simulink model "final"  (R2020a)
settings: Solver=VariableStepAuto  StartTime=0.0  StopTime=5  RelTol=1e-3
undefined symbols (not defined in the file): fdesignblkfcn, gcbh
libraries: dspvision x6, dspfdesign x2, audiosources x1, dspsnks4 x1, dsparch4 x1, dspsrcs4 x1
settings Model: Creator=Karan  LastModifiedBy=Karan

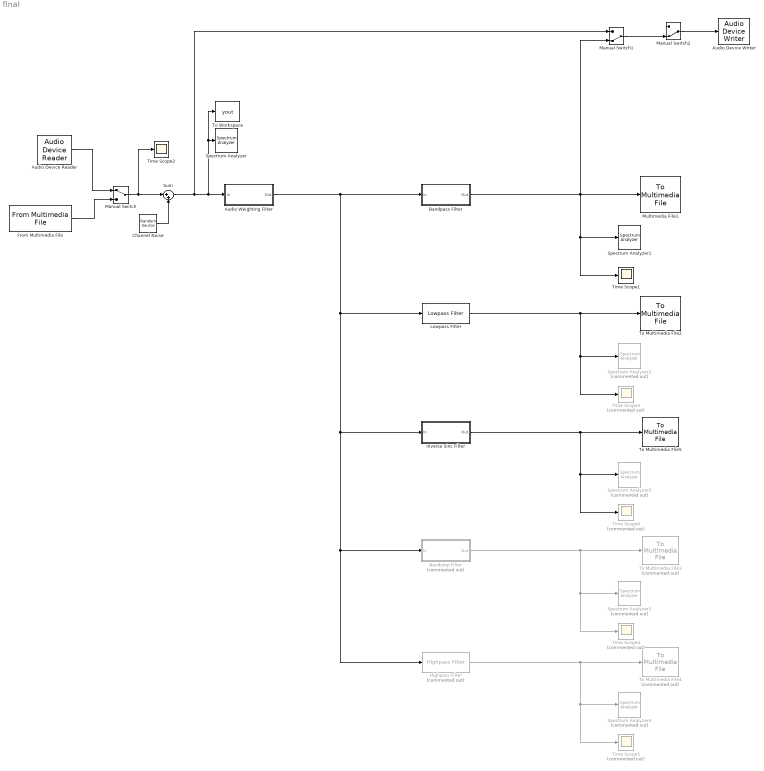
== system final ==
  Audio Device Reader : audiosources/Audio Device Reader  Driver=DirectSound  Device=Default  SampleRate=44100  NumChannels=1  SamplesPerFrame=1024  BitDepth=16-bit integer  NumBuffers=10  DefaultInputChannelMapping=on  InputChannelMapping=1:2  OutputNumOverrunSamples=off  OutputDataType=double  DriverIdx=1  DeviceWarnFlag=''
      settings: SourceProductBaseCode=AU
  Audio Device Writer : dspsnks4/Audio Device Writer  Driver=DirectSound  Device=Default  InheritSampleRate=on  SampleRate=44100  BitDepth=16-bit integer  BufferSize=4096  NumBuffers=10  DefaultOutputChannelMapping=on  OutputChannelMapping=1:2  OutputNumUnderrunSamples=off  DriverIdx=1  DeviceWarnFlag=''
  Audio Weighting Filter : Subsystem  DialogController=fdesignblkfcn  InitFcn=fdesignblkfcn(gcbh, {'InitFcn'});  mask(Audio Weighting Filter){}
      mask help: Design an audio weighting filter
      settings: CopyFcn=fdesignblkfcn(gcbh, {'CopyFcn'});
      mask Help: helpview(mapfilelocation('dsp'), 'dspaudioweightingfilter');
      mask Display: disp('Audio Weighting')
  Bandpass Filter : Subsystem  DialogController=fdesignblkfcn  InitFcn=fdesignblkfcn(gcbh, {'InitFcn'});  mask(Bandpass Filter){}
      mask help: Design a bandpass filter
      settings: CopyFcn=fdesignblkfcn(gcbh, {'CopyFcn'});
      mask Help: helpview(mapfilelocation('dsp'), 'dspbandpassfilter');
      mask Display: disp('Bandpass');
  Bandstop Filter : Subsystem  Commented=on  DialogController=fdesignblkfcn  InitFcn=fdesignblkfcn(gcbh, {'InitFcn'});  mask(Bandstop Filter){}
      mask help: Design a bandstop filter
      settings: CopyFcn=fdesignblkfcn(gcbh, {'CopyFcn'});
      mask Help: helpview(mapfilelocation('dsp'), 'dspbandstopfilter');
      mask Display: disp('Bandstop');
  Channel Noise : dspsrcs4/Random Source  SrcType=Gaussian  NormMethod=Ziggurat  CltLength=12  MinVal=0  MaxVal=1  MeanVal=0  VarVal=0.000005  RepMode=Not repeatable  rawSeed=1  IsInherit=off  SampMode=Discrete  SampTime=1/44100  SampFrame=1024  DataType=Double  OutComplex=Real  OutputFrames=off
  From Multimedia File : dspvision/From Multimedia File  inputFilename=D:\projects_on_github\tri-8_project\Matlab\dataset\noisy1.wav  readRange=[1 Inf]  loop=on  numPlays=inf  outputStreams=Audio only  videoDataType=single  audioDataType=double  inheritSampleTime=on  userDefinedSampleTime=1/30  noAudioOutput=off  isIntensityVideo=off  fourcc=RGB  colorVideoFormat=Separate color signals  outputEOF=off  dataOrg=Column-major  audioFrameSize=1024  computeAudioFrameSize=off  outSamplingMode=Sample based
  Highpass Filter : dspfdesign/Highpass Filter  Commented=on  FilterType=FIR  DesignForMinimumOrder=on  FilterOrder=50  StopbandFrequency=8e3  PassbandFrequency=12e3  StopbandAttenuation=80  PassbandRipple=0.1  InheritSampleRate=off  SampleRate=44100  SimulateUsing=Interpreted execution  roundingMode=Floor  coeffsDataTypeStr=fixdt(1,16)
  Inverse Sinc Filter : Subsystem  DialogController=fdesignblkfcn  InitFcn=fdesignblkfcn(gcbh, {'InitFcn'});  mask(Inverse Sinc Filter){}
      mask help: Design an inverse sinc filter
      settings: CopyFcn=fdesignblkfcn(gcbh, {'CopyFcn'});
      mask Help: helpview(mapfilelocation('dsp'), 'dspinversesincfilter');
      mask Display: disp('Inverse Sinc');
  Lowpass Filter : dspfdesign/Lowpass Filter  FilterType=FIR  DesignForMinimumOrder=on  FilterOrder=50  PassbandFrequency=3400  StopbandFrequency=6000  PassbandRipple=0.1  StopbandAttenuation=80  InheritSampleRate=off  SampleRate=44100  SimulateUsing=Interpreted execution  roundingMode=Floor  coeffsDataTypeStr=fixdt(1,16)
  Manual Switch : ManualSwitch
  Manual Switch1 : ManualSwitch  CurrentSetting=0
  Manual Switch2 : ManualSwitch  CurrentSetting=0
  Multimedia File1 : dspvision/To Multimedia File  outputFilename=D:\projects_on_github\tri-8_project\Matlab\BandPassOutput.wav  streamSelection=Audio only  videoCompressor=None (uncompressed)  audioCompressor=None (uncompressed)  imagePorts=Separate color signals  fileType=WAV  audioDatatype=16-bit integer  fourcc=RGB  videoQuality=75  mj2000CompFactor=10  mask(To Multimedia File){}
      mask Display: image('D:\projects_on_github\tri-8_project\icon.jfif'); % Use "Edit Image" on toolstrip to change.
  Spectrum Analyzer : SpectrumAnalyzer
  Spectrum Analyzer1 : SpectrumAnalyzer
  Spectrum Analyzer{2..5} (4 alike) : SpectrumAnalyzer  Commented=on
  Sum : Sum  Inputs=|++
  Time Scope1 : Scope
  Time Scope2 : Scope
  Time Scope{3..6} (4 alike) : Scope  Commented=on
  To Multimedia File2 : dspvision/To Multimedia File  outputFilename=D:\projects_on_github\tri-8_project\Matlab\LowPassOutput.wav  streamSelection=Audio only  videoCompressor=None (uncompressed)  audioCompressor=None (uncompressed)  imagePorts=Separate color signals  fileType=WAV  audioDatatype=16-bit integer  fourcc=RGB  videoQuality=75  mj2000CompFactor=10  mask(To Multimedia File){}
      mask Display: image('D:\projects_on_github\tri-8_project\icon.jfif'); % Use "Edit Image" on toolstrip to change.
  To Multimedia File3 : dspvision/To Multimedia File  Commented=on  outputFilename=D:\projects_on_github\tri-8_project\Matlab\BandStopOutput.wav  streamSelection=Audio only  videoCompressor=None (uncompressed)  audioCompressor=None (uncompressed)  imagePorts=Separate color signals  fileType=WAV  audioDatatype=16-bit integer  fourcc=RGB  videoQuality=75  mj2000CompFactor=10
  To Multimedia File4 : dspvision/To Multimedia File  Commented=on  outputFilename=D:\projects_on_github\tri-8_project\Matlab\HighPassOutput.wav  streamSelection=Audio only  videoCompressor=None (uncompressed)  audioCompressor=None (uncompressed)  imagePorts=Separate color signals  fileType=WAV  audioDatatype=16-bit integer  fourcc=RGB  videoQuality=75  mj2000CompFactor=10
  To Multimedia File5 : dspvision/To Multimedia File  outputFilename=D:\projects_on_github\tri-8_project\Matlab\InverseSincOutput.wav  streamSelection=Audio only  videoCompressor=None (uncompressed)  audioCompressor=None (uncompressed)  imagePorts=Separate color signals  fileType=WAV  audioDatatype=16-bit integer  fourcc=RGB  videoQuality=75  mj2000CompFactor=10  mask(To Multimedia File){}
      mask Display: image('D:\projects_on_github\tri-8_project\icon.jfif'); % Use "Edit Image" on toolstrip to change.
  To Workspace : ToWorkspace  VariableName=yout  SampleTime=-1
      settings: Save2DSignal=2-D array (concatenate along first dimension)
  wires:
  From Multimedia File/1 -> Manual Switch/2
  Audio Device Reader/1 -> Manual Switch/1
  Channel Noise/1 -> Sum/2
  Manual Switch/1 -> Time Scope2/1, Sum/1
  Lowpass Filter/1 -> Spectrum Analyzer2/1, Time Scope3/1, To Multimedia File2/1
  Bandstop Filter/1(Out) -> Spectrum Analyzer3/1, Time Scope4/1, To Multimedia File3/1
  Highpass Filter/1 -> Spectrum Analyzer4/1, Time Scope5/1, To Multimedia File4/1
  Sum/1 -> Manual Switch1/1, Audio Weighting Filter/1(In), To Workspace/1, Spectrum Analyzer/1
  Audio Weighting Filter/1(Out) -> Highpass Filter/1, Bandstop Filter/1(In), Inverse Sinc Filter/1(In), Lowpass Filter/1, Bandpass Filter/1(In)
  Bandpass Filter/1(Out) -> Manual Switch1/2, Multimedia File1/1, Spectrum Analyzer1/1, Time Scope1/1
  Inverse Sinc Filter/1(Out) -> Spectrum Analyzer5/1, Time Scope6/1, To Multimedia File5/1
  Manual Switch1/1 -> Manual Switch2/2
  Manual Switch2/1 -> Audio Device Writer/1

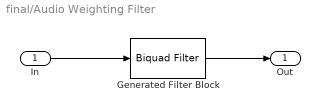
== system final/Audio Weighting Filter ==
  In : Inport
  Generated Filter Block : dsparch4/Biquad Filter  Tag=BlockMethodSubSystem  FilterSource=Dialog parameters  CoeffSource=Specify via dialog  FilterObject=BQF  IIRFiltStruct=Direct form II  BiQuadCoeffs=[0.000322318592897718971 0.000644637185795437942 0.000322318592897718971 1 -0.22455845805977917 0.0126066252715463997;1 -2 1 1 -1.89387049472307045 0.895159769094661439;1 -2 1 1 -1.99461445599302167 0.994621707014084477]  ScaleValues=[0.788048167211767292;1;1;922.43864463225691]  IC=0  ICnum=0  ICden=0  a0Flag=Warning  optimizeScaleValues=off  ScaleValueMode=Specify via input port (g)  InputProcessing=Columns as channels (frame based)  roundingMode=Floor  overflowMode=off  scaleValueFracLength=14  denProdOutputFracLength=30  denAccumFracLength=30  secondMemoryFracLength=15
  Out : Outport  VectorParamsAs1DForOutWhenUnconnected=off
  wires:
  In/1 -> Generated Filter Block/1
  Generated Filter Block/1 -> Out/1

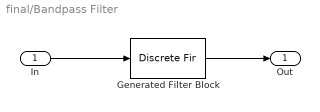
== system final/Bandpass Filter ==
  In : Inport
  Generated Filter Block : DiscreteFir  Tag=BlockMethodSubSystem  Coefficients=[-0.000844527152407708605 -0.000868562397225502948 -0.00116957293952449923 -0.00140352553207754964 -0.00150744965775681137 -0.00142845443379888918 -0.00113615100032245946 -0.000633399920489026349 3.8890998282847068e-05 0.000802430669925044394 0.00155053327984106849 0.00216334568785815553 0.00252906066623926869 0.00256430053522338887 0.0022313474523283929 0.00154779936195130279 0.000589010105671559014 -0.000522288015542289445 -0.00163619716288358297 -0.00260090540526047896 -0.00328662298843564573 -0.00361236887478878299 -0.00356005546849189926 -0.00317324951512466553 -0.00255473905797780603 -0.00183884524741045039 -0.00116989216351721611 -0.0006702717355624154 -0.000417805025534387635 -0.000430709163936836151 -0.000666023921114739566 -0.00103063604797135012 -0.00140285309979080227 -0.00166073040719528597 -0.00170975104047725937 -0.00150416142672811178 -0.00105705997801263459 -0.00043816865408110358 0.000242513896455011108 0.000859775723202255908 0.00130153535695951244 0.00149428225464512919 0.00142096258781483132 0.00112380329738751895 0.000695630323721911723 0.000258307321682619661 -6.65169364834449476e-05 -0.000184471009694367179 -5.22502422152739231e-05 0.000312808959320525664 0.000835725379946367281 0.00140171113245306581 0.00188290629102422571 0.0021687101586182209 0.00219279555742255905 0.00194960550536461309 0.0014967883978339602 0.000942467091606558711 0.000420688844749388829 5.9455733870843644e-05 -4.95874098292944614e-05 0.00012611843689524363 0.000551229383838804468 0.00112968550315262705 0.00172705058986454625 0.00220135626888997779 0.00243796013325304085 0.00237723221351059414 0.0020301515849451765 0.00147739859898147878 0.000851134737987892936 0.000304645405197287596 -2.45362664157255234e-05 -4.78931844306208036e-05 0.000251503798032808382 0.000813143385485723424 0.00151197185459038975 0.00218687423025305588 0.00267876041303893994 0.00286884600272527008 0.0027084843946502562 0.00223220324906475091 0.00155177460699580162 0.000830826586767605645 0.000246619686949600561 -5.25568822962958e-05 1.62854310485545643e-05 0.000448608883877401037 0.00115176008790661877 0.00196461380074925687 0.00269513061748809582 0.00316573559661484502 0.00325667292570079201 0.00293645872877977771 0.00227166552482126888 0.00141343803054731982 0.00056310351191782564 -7.53025250680251833e-05 -0.000344157009495414049 -0.000171780476247792164 0.000408022839556828969 0.0012612403531024061 0.00218361284411515595 0.00294781870362859685 0.00335822952789425208 0.00329883802248306891 0.00276364882401694805 0.00186096741407613042 0.000790494870982292133 -0.000202827515527535443 -0.000886470403153027551 -0.00109739540988425168 -0.000783030915458725958 -1.73930802721871426e-05 0.0010136082637835107 0.00205387967773256125 0.00283728196811974982 0.00315177869803649063 0.00289235940759398607 0.0020893396216802528 0.000905051665350609926 -0.000401866909465046639 -0.00153626562781204105 -0.00223704372134110553 -0.00234118477513825833 -0.00182637015731584949 -0.00082014067502192943 0.000426324760092775402 0.00159568661965235983 0.00237922054570370491 0.00255207910415520406 0.00203002271684176025 0.000894367368082263532 -0.000623077482255825644 -0.00219127628456664524 -0.00345756871074918851 -0.00413211362214908375 -0.00406036258673411754 -0.00326452265175293781 -0.0019437873571267225 -0.000431420107182345965 0.000881658006659412829 0.00164005892403595562 0.00161107111147124451 0.000745200775659432958 -0.000805996364953532034 -0.00271994083762002164 -0.00457588016984548755 -0.00595336149238870956 -0.00653452096578667051 -0.00618437479048854124 -0.00498998409671571816 -0.00324668708151827287 -0.00139387104974101109 8.68820925025471931e-05 0.000786909783874334824 0.000472575305548095486 -0.000852098204424628293 -0.00293738456659842391 -0.00533975824108989198 -0.00752207712372473473 -0.00898062826097165146 -0.00936845343587668078 -0.00858577816341373271 -0.00681354149649567205 -0.00448070355246299803 -0.00216977611076906406 -0.000481692636351701133 ...(+6520 chars)]  InputProcessing=Columns as channels (frame based)
  Out : Outport  VectorParamsAs1DForOutWhenUnconnected=off
  wires:
  In/1 -> Generated Filter Block/1
  Generated Filter Block/1 -> Out/1

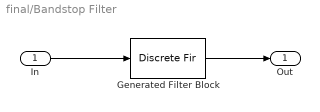
== system final/Bandstop Filter ==
  In : Inport
  Generated Filter Block : DiscreteFir  Tag=BlockMethodSubSystem  Coefficients=[-0.00049984690227566171 9.5100318056220678e-05 -0.018778888889125381 0.00020561736622238936 0.0019605411941885044 0.00023848464356614288 0.011427768692370117 0.00024928020776728103 -0.026344143468356181 0.00022323473160311075 0.033802321854574921 0.00024455404571586617 -0.019823660150560137 0.00024377045334422507 -0.019896328302992174 0.00022786848806407702 0.082714162332194516 0.00025656261277749384 -0.15101859373266049 0.00022072984516862497 0.20526035643478094 0.0002476136866061962 0.77489283142488197 0.0002476136866061962 0.20526035643478094 0.00022072984516862497 -0.15101859373266049 0.00025656261277749384 0.082714162332194516 0.00022786848806407702 -0.019896328302992174 0.00024377045334422507 -0.019823660150560137 0.00024455404571586617 0.033802321854574921 0.00022323473160311075 -0.026344143468356181 0.00024928020776728103 0.011427768692370117 0.00023848464356614288 0.0019605411941885044 0.00020561736622238936 -0.018778888889125381 9.5100318056220678e-05 -0.00049984690227566171]  InputProcessing=Columns as channels (frame based)
  Out : Outport  VectorParamsAs1DForOutWhenUnconnected=off
  wires:
  Generated Filter Block/1 -> Out/1
  In/1 -> Generated Filter Block/1

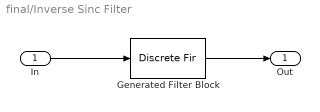
== system final/Inverse Sinc Filter ==
  In : Inport
  Generated Filter Block : DiscreteFir  Tag=BlockMethodSubSystem  Coefficients=[-0.000928481225776401362 -0.000685248099900260545 0.000396415563561522649 0.0031279119219253769 0.00745022627781007519 0.0123212966122183253 0.0157155430609445569 0.0151746343302536554 0.00886627464558614915 -0.00320567481684330387 -0.0183661889719039621 -0.0313404653493913679 -0.0354651834927562706 -0.0248237025198619517 0.00336517479562531288 0.047033122810189204 0.0989991274361954887 0.148484198098675746 0.184043034456273541 0.196976246131404104 0.184043034456273541 0.148484198098675746 0.0989991274361954887 0.047033122810189204 0.00336517479562531288 -0.0248237025198619517 -0.0354651834927562706 -0.0313404653493913679 -0.0183661889719039621 -0.00320567481684330387 0.00886627464558614915 0.0151746343302536554 0.0157155430609445569 0.0123212966122183253 0.00745022627781007519 0.0031279119219253769 0.000396415563561522649 -0.000685248099900260545 -0.000928481225776401362]  InputProcessing=Columns as channels (frame based)
  Out : Outport  VectorParamsAs1DForOutWhenUnconnected=off
  wires:
  Generated Filter Block/1 -> Out/1
  In/1 -> Generated Filter Block/1
